simulink model "motorcycle_simulink_with_integral_action"  (R2021a)
settings: Solver=VariableStepAuto  StartTime=0.0  StopTime=10  RelTol=1e-3
settings Model: Creator=martina.elle  LastModifiedBy=francesco

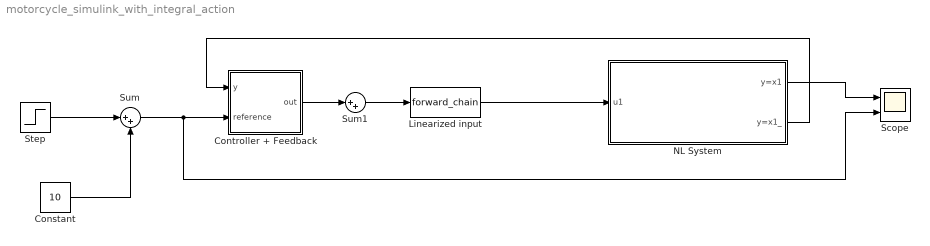
== system motorcycle_simulink_with_integral_action ==
  Constant : Constant  Value=10
  Controller + Feedback : Subsystem
  "Linearized input " : MATLABFcn  MATLABFcn=forward_chain  OutputDimensions=1
  NL System : Subsystem
  Scope : Scope  NumInputPorts=2
  Step : Step  SampleTime=0
  Sum : Sum  Inputs=|++
  Sum1 : Sum  Inputs=|++
  wires:
  "Linearized input "/1 -> NL System/1(u1)
  NL System/2(y=x1_) -> Controller + Feedback/1(y)
  NL System/1(y=x1) -> Scope/1
  Step/1 -> Sum/1
  Constant/1 -> Sum/2
  Sum/1 -> Scope/2, Controller + Feedback/2(reference)
  Controller + Feedback/1(out) -> Sum1/1
  Sum1/1 -> "Linearized input "/1

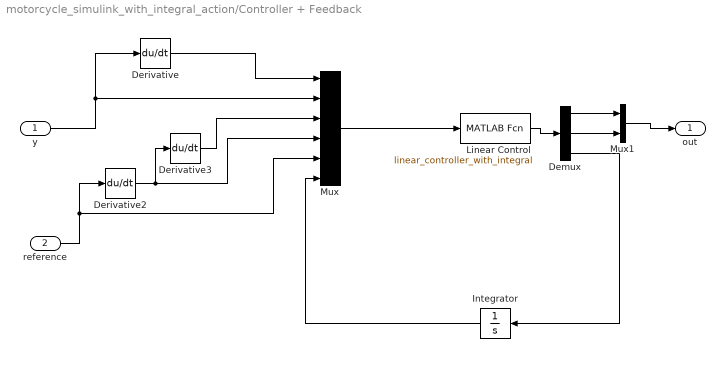
== system motorcycle_simulink_with_integral_action/Controller + Feedback ==
  y : Inport
  reference : Inport  Port=2
  Demux : Demux  Outputs=3
  Derivative : Derivative
  Derivative2 : Derivative
  Derivative3 : Derivative
  Integrator : Integrator  InitialCondition=1
  Linear Control : MATLABFcn  MATLABFcn=linear_controller_with_integral  OutputDimensions=3
  Mux : Mux  Inputs=6
  Mux1 : Mux  Inputs=2
  out : Outport
  wires:
  y/1 -> Derivative/1, Mux/2
  reference/1 -> Mux/5, Derivative2/1
  Derivative2/1 -> Mux/4, Derivative3/1
  Derivative/1 -> Mux/1
  Derivative3/1 -> Mux/3
  Mux/1 -> Linear Control/1
  Demux/1 -> Mux1/1
  Demux/2 -> Mux1/2
  Mux1/1 -> out/1
  Linear Control/1 -> Demux/1
  Demux/3 -> Integrator/1
  Integrator/1 -> Mux/6

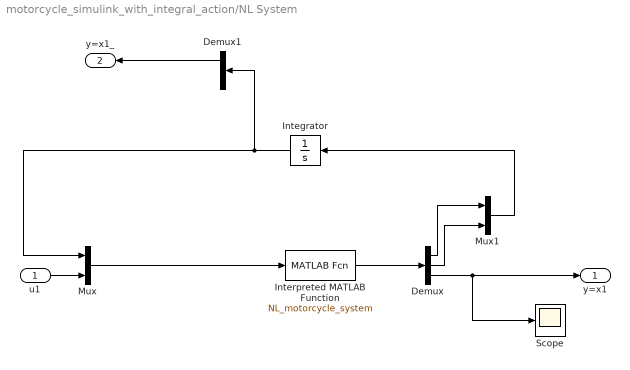
== system motorcycle_simulink_with_integral_action/NL System ==
  u1 : Inport
  Demux : Demux  Outputs=3
  Demux1 : Demux  Outputs=2
  Integrator : Integrator  InitialCondition=[10 10]
  Interpreted MATLAB Function : MATLABFcn  MATLABFcn=NL_motorcycle_system  OutputDimensions=3
  Mux : Mux  Inputs=2
  Mux1 : Mux  Inputs=2
  Scope : Scope
  y=x1 : Outport
  y=x1_ : Outport  Port=2
  wires:
  u1/1 -> Mux/2
  Demux/2 -> Mux1/2
  Mux/1 -> Interpreted MATLAB Function/1
  Mux1/1 -> Integrator/1
  Integrator/1 -> Demux1/1, Mux/1
  Demux/1 -> Mux1/1
  Interpreted MATLAB Function/1 -> Demux/1
  Demux/3 -> Scope/1, y=x1/1
  Demux1/1 -> y=x1_/1
